simulink model "Simulin5"  (R2024b)
settings: Solver=FixedStepAuto  StartTime=0.0  StopTime=0.250  FixedStep=0.00001  RelTol=1e-3
values from neighbouring files (symbols this model uses):
  Kd = 0.001    [Prac5.m]
  Ki = 1000    [Prac5.m]
  Kp = 10    [Prac5.m]
libraries: slpidlib x1
settings Model: Creator=PROBOOK  LastModifiedBy=PROBOOK

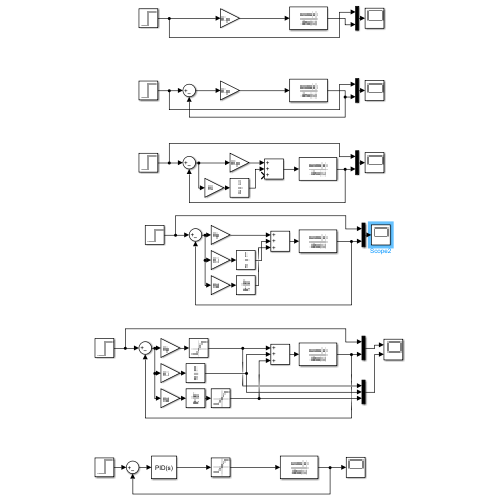
[thumbnail: Simulink's stored preview of the top-level diagram]
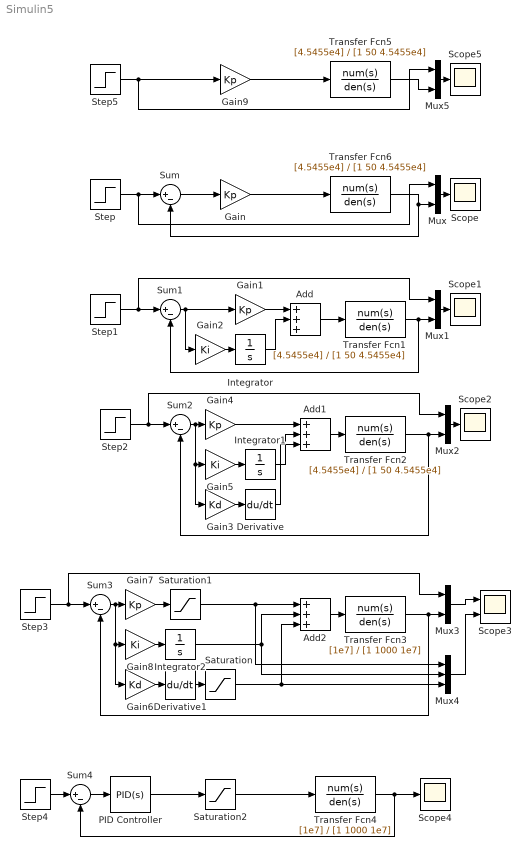
== system Simulin5 ==
  Add : Sum  Inputs=+++
  Add1 : Sum  Inputs=+++
  Add2 : Sum  Inputs=+++
  Derivative : Derivative
  Derivative1 : Derivative
  Gain{,1,4,7,9} (5 alike) : Gain  Gain=Kp
  Gain2 : Gain  Gain=Ki
  Gain3 : Gain  Gain=Kd
  Gain5 : Gain  Gain=Ki
  Gain6 : Gain  Gain=Kd
  Gain8 : Gain  Gain=Ki
  Integrator : Integrator
  Integrator1 : Integrator
  Integrator2 : Integrator
  Mux{,1..3,5} (5 alike) : Mux  Inputs=2
  Mux4 : Mux  Inputs=3
  PID Controller : slpidlib/PID Controller  Controller=PID  Form=Parallel  TimeDomain=Continuous-time  UseExternalTs=off  SampleTime=-1  IntegratorMethod=Forward Euler  FilterMethod=Forward Euler  ControllerParametersSource=internal  P=0  I=10.0576853561284  UseKiTs=off  D=0  UseExternalDerivativeSource=off  N=100  UseFilter=on  TunerSelectOption=Transfer Function Based (PID Tuner App)  InitialConditionSource=internal  InitialConditionForIntegrator=0  InitialConditionForFilter=0  DifferentiatorICPrevScaledInput=0  ExternalReset=none  TrackingMode=off  Kt=1  LimitOutput=off  SatLimitsSource=internal  UpperSaturationLimit=inf  LowerSaturationLimit=-inf  LinearizeAsGain=on  AntiWindupMode=external  Kb=1  LimitIntegrator=off  UpperIntegratorSaturationLimit=inf  LowerIntegratorSaturationLimit=-inf  POutMin=[]  POutMax=[]  IOutMin=[]  IOutMax=[]  DOutMin=[]  DOutMax=[]  NOutMin=[]  NOutMax=[]  SumOutMin=[]  SumOutMax=[]  SaturationOutMin=[]  SaturationOutMax=[]  PParamMin=[]  PParamMax=[]  IParamMin=[]  IParamMax=[]  DParamMin=[]  DParamMax=[]  NParamMin=[]  NParamMax=[]  KbParamMin=[]  KbParamMax=[]  KtParamMin=[]  KtParamMax=[]  KbOutMin=[]  KbOutMax=[]  KtOutMin=[]  KtOutMax=[]  IntegratorOutMin=[]  IntegratorOutMax=[]  FilterOutMin=[]  FilterOutMax=[]  SumI1OutMin=[]  SumI1OutMax=[]  SumI2OutMin=[]  SumI2OutMax=[]  SumI3OutMin=[]  SumI3OutMax=[]  SumI4OutMin=[]  SumI4OutMax=[]  SumDOutMin=[]  SumDOutMax=[]  DifferentiatorOutMin=[]  DifferentiatorOutMax=[]  FilterDiffOutCoefMin=[]  FilterDiffOutCoefMax=[]  ReciprocalOutMin=[]  ReciprocalOutMax=[]  SumDenOutMin=[]  SumDenOutMax=[]  SumNumOutMin=[]  SumNumOutMax=[]  DivideOutMin=[]  DivideOutMax=[]  UdiffTsProdOutMin=[]  UdiffTsProdOutMax=[]  NTsProdOutMin=[]  NTsProdOutMax=[]  UintegralTsProdOutMin=[]  UintegralTsProdOutMax=[]  UngainTsProdOutMin=[]  UngainTsProdOutMax=[]  ClampingZeroOutDataTypeStr=Inherit: Inherit via back propagation  ClampingZeroOutMin=[]  ClampingZeroOutMax=[]  FilterDenConstantOutDataTypeStr=Inherit: Inherit via back propagation  FilterDenConstantOutMin=[]  FilterDenConstantOutMax=[]  PCopyOutDataTypeStr=Inherit: Inherit via back propagation  PCopyOutMin=[]  PCopyOutMax=[]  NCopyOutDataTypeStr=Inherit: Inherit via back propagation  NCopyOutMin=[]  NCopyOutMax=[]  IntegratorContinuousStateAttributes=''  IntegratorStateMustResolveToSignalObject=off  IntegratorRTWStateStorageClass=Auto  FilterContinuousStateAttributes=''  FilterStateMustResolveToSignalObject=off  FilterRTWStateStorageClass=Auto  ParallelPVariant=InternalParameters  IdealPVariant=Disabled  IVariant=InternalParameters  DVariant=InternalParameters  IntegratorVariant=Continuous  SatVariant=Disabled  AWVariant=Passthrough  PCopyVariant=Disabled  TRVariant=Disabled  FdbkBlocksVariant=Forward  IdealPFdbkVariant=Disabled  SatFdbkVariant=Disabled  DerivativeFilterVariant=ContFilter  NVariant=InternalParameters  NCopyVariant=Disabled  FilterICVariant=InternalICsFilter  IntegratorICVariant=InternalICs  ExternalResetVariant=Disabled  TRSumVariant=Passthrough  SumFdbkVariant=Disabled  SumVariant=Sum_PID  TsampFilterVariant=InternalTs  TsampNgainVariant=Passthrough  TsampIntegralVariant=Disabled_SignalSpec  ExternalSaturationOutDataTypeStr=Inherit: Same as second input  DerivativeSourceVariant=ErrorSignal  PreIntVariant=InternalPreInt
  Saturation : Saturate  UpperLimit=15  LowerLimit=-15
  Saturation1 : Saturate
  Saturation2 : Saturate  UpperLimit=15  LowerLimit=-15
  Scope{,1..2,4..5} (5 alike) : Scope
  Scope3 : Scope  NumInputPorts=2
  Step : Step  Time=0.01  After=5  SampleTime=0
  Step{1..4} (4 alike) : Step  Time=0.01  SampleTime=0
  Step5 : Step  Time=0.01  After=5  SampleTime=0
  Sum{,1..4} (5 alike) : Sum  Inputs=|+-
  Transfer Fcn{1..2,5..6} (4 alike) : TransferFcn  Numerator=[4.5455e4]  Denominator=[1 50 4.5455e4]
  Transfer Fcn3 : TransferFcn  Numerator=[1e7]  Denominator=[1 1000 1e7]
  Transfer Fcn4 : TransferFcn  Numerator=[1e7]  Denominator=[1 1000 1e7]
  wires:
  Step/1 -> Mux/1, Sum/1
  Sum/1 -> Gain/1
  Gain/1 -> Transfer Fcn6/1
  Transfer Fcn6/1 -> Mux/2, Sum/2
  Mux/1 -> Scope/1
  Transfer Fcn1/1 -> Mux1/2, Sum1/2
  Step1/1 -> Mux1/1, Sum1/1
  Sum1/1 -> Gain2/1, Gain1/1
  Gain1/1 -> Add/1
  Gain2/1 -> Integrator/1
  Integrator/1 -> Add/2
  Mux1/1 -> Scope1/1
  Add/1 -> Transfer Fcn1/1
  Integrator1/1 -> Add1/2
  Gain5/1 -> Integrator1/1
  Add1/1 -> Transfer Fcn2/1
  Gain4/1 -> Add1/1
  Mux2/1 -> Scope2/1
  Transfer Fcn2/1 -> Mux2/2, Sum2/2
  Step2/1 -> Mux2/1, Sum2/1
  Sum2/1 -> Gain3/1, Gain5/1, Gain4/1
  Derivative/1 -> Add1/3
  Gain3/1 -> Derivative/1
  Gain6/1 -> Derivative1/1
  Mux3/1 -> Scope3/1
  Add2/1 -> Transfer Fcn3/1
  Transfer Fcn3/1 -> Mux3/2, Sum3/2
  Step3/1 -> Mux3/1, Sum3/1
  Gain8/1 -> Integrator2/1
  Integrator2/1 -> Add2/2, Mux4/2
  Sum3/1 -> Gain6/1, Gain8/1, Gain7/1
  Derivative1/1 -> Saturation/1
  Saturation/1 -> Add2/3, Mux4/3
  Gain7/1 -> Saturation1/1
  Saturation1/1 -> Mux4/1, Add2/1
  Mux4/1 -> Scope3/2
  Transfer Fcn4/1 -> Sum4/2, Scope4/1
  PID Controller/1 -> Saturation2/1
  Saturation2/1 -> Transfer Fcn4/1
  Step4/1 -> Sum4/1
  Sum4/1 -> PID Controller/1
  Transfer Fcn5/1 -> Mux5/2
  Gain9/1 -> Transfer Fcn5/1
  Mux5/1 -> Scope5/1
  Step5/1 -> Gain9/1, Mux5/1
